simulink model "inverter"  (Simulink 3.00)
settings: Solver=ode4  StartTime=0.0  StopTime=0.05  FixedStep=1e-6  MaxStep=1e-4
libraries: simulink3 x1
settings Model: Refine=3  SaveTime=off  TimeSaveName=t  SaveOutput=off  OutputSaveName=y

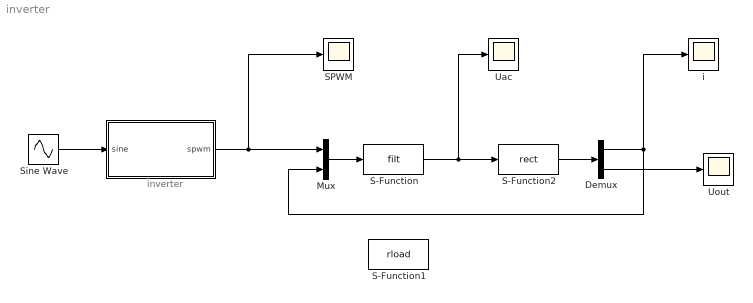
== system inverter ==
  note: inverter
  " " : Subsystem
  Demux : Demux  Outputs=2
  Mux : Mux  Inputs=2
  S-Function : S-Function  FunctionName=filt  Parameters=0.528e-3,300e-6,44e-6,1  PortCounts=[]  SFunctionModules=''
  S-Function1 : S-Function  FunctionName=rload  Parameters=50  PortCounts=[]  SFunctionModules=''
  S-Function2 : S-Function  FunctionName=rect  Parameters=1,4700e-6,50  PortCounts=[]  SFunctionModules=''
  SPWM : Scope
      settings: TimeRange=0.05  YMin=-250  YMax=250  SaveToWorkspace=off  SaveName=ScopeData  LimitMaxRows=off
  Sine Wave : Sin  Amplitude=4  Frequency=800*pi  Phase=0  SampleTime=0
  Uac : Scope
      settings: TimeRange=0.01  YMin=-200  YMax=200  SaveToWorkspace=off  SaveName=ScopeData  LimitMaxRows=off
  Uout : Scope
      settings: TimeRange=0.05  YMin=-200  YMax=200  SaveToWorkspace=off  SaveName=ScopeData  LimitMaxRows=off
  i : Scope
      settings: TimeRange=0.05  YMin=-60  YMax=50  SaveToWorkspace=off  SaveName=ScopeData  LimitMaxRows=off
  wires:
  Sine Wave/1 -> " "/1(sine)
  Mux/1 -> S-Function/1
  S-Function2/1 -> Demux/1
  Demux/2 -> Uout/1
  S-Function/1 -> Uac/1, S-Function2/1
  " "/1(spwm) -> Mux/1, SPWM/1
  Demux/1 -> i/1, Mux/2

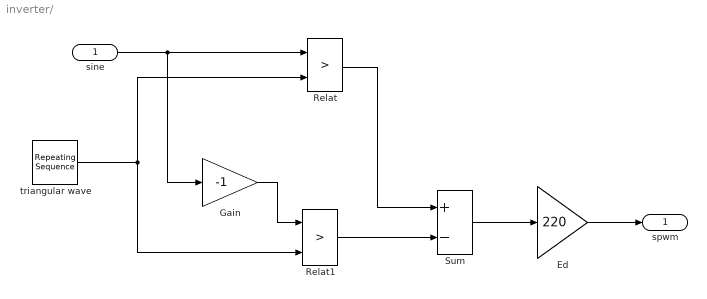
== system inverter/  ==
  sine : Inport  Port=1  PortWidth=-1  SampleTime=-1  DataType=auto
      settings: SignalType=auto
  Ed : Gain  Gain=220  SaturateOnIntegerOverflow=on
  Gain : Gain  Gain=-1  SaturateOnIntegerOverflow=on
  Relat : RelationalOperator  Operator=>
  Relat1 : RelationalOperator  Operator=>
  Sum : Sum  Inputs=+-  SaturateOnIntegerOverflow=on
  triangular wave : simulink3/Sources/Repeating Sequence  rep_seq_t=[0 1/48e3 1/16e3 1/12e3]  rep_seq_y=[0 5 -5 0]
  spwm : Outport  Port=1
  wires:
  Sum/1 -> Ed/1
  sine/1 -> Relat/1, Gain/1
  Gain/1 -> Relat1/1
  triangular wave/1 -> Relat/2, Relat1/2
  Ed/1 -> spwm/1
  Relat/1 -> Sum/1
  Relat1/1 -> Sum/2
